simulink model "Model-Reglare"  (R2021b)
settings: Solver=ode45  StartTime=0.0  StopTime=1000  RelTol=1e-3  EnableMultiTasking=on
undefined symbols (not defined in the file): k, k1, k11, k12, k13, k2, k3, keta
libraries: slpidlib x8
(part 1 of 2)
settings Model: Creator=Nicoleta  LastModifiedBy=daria.chiriac
settings SolverCC: AlgebraicLoopSolver=TrustRegion
settings DataIOCC: LimitDataPoints=on  SaveFormat=Array  ReturnWorkspaceOutputs=off
settings OptimizationCC: LifeSpan=inf
settings DebuggingCC: SFUnexpectedBacktrackingDiag=warning  SFNoUnconditionalDefaultTransitionDiag=warning  SFExecutionAtInitializationDiag=none  SFMachineParentedDataDiag=warning  ArithmeticOperatorsInVariantConditions=warning
settings HardwareCC: ProdBitPerPointer=32  ProdBitPerSizeT=32  ProdBitPerPtrDiffT=32  ProdLargestAtomicFloat=None  ProdIntDivRoundTo=Undefined  ProdEndianess=Unspecified  ProdWordSize=32  ProdHWDeviceType=32-bit Generic
settings ModelReferenceCC: PropagateSignalLabelsOutOfModel=off
settings SFSimCC: SimUseLocalCustomCode=off  CustomCodeUndefinedFunction=UseInterfaceOnly
settings RTWCC: RTWUseLocalCustomCode=off
settings CodeAppCC: StateflowObjectComments=on
settings GRTTargetCC: TargetLangStandard=C89/C90 (ANSI)
settings ConfigComp: CovMetricSettings=dw  CovSaveCumulativeToWorkspaceVar=on  CovSaveSingleToWorkspaceVar=on  CovExternalEMLEnable=off

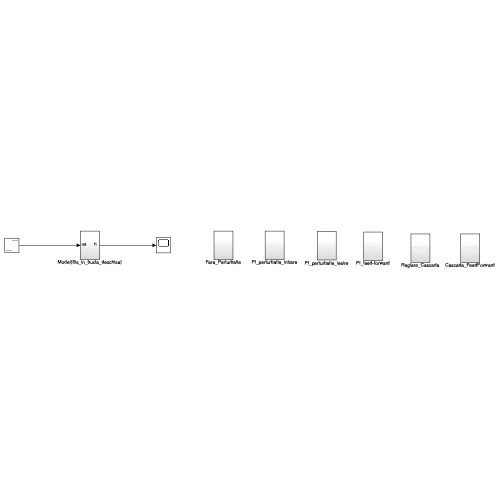
[thumbnail: Simulink's stored preview of the top-level diagram]
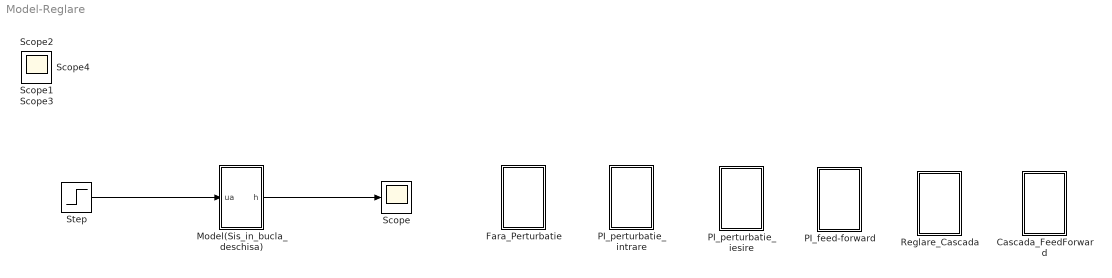
== system Model-Reglare ==
  Cascada_FeedForward : Subsystem
  Fara_Perturbatie : Subsystem
  Model(Sis_in_bucla_deschisa) : Subsystem
  PI_feed-forward : Subsystem
  PI_perturbatie_iesire : Subsystem
  PI_perturbatie_intrare : Subsystem
  Reglare_Cascada : Subsystem
  Scope{,1..4} (5 alike) : Scope
  Step : Step  After=5  SampleTime=0
  wires:
  Model(Sis_in_bucla_deschisa)/1("h ") -> Scope/1
  Step/1 -> Model(Sis_in_bucla_deschisa)/1("ua ")

== system Model-Reglare/Cascada_FeedForward ==
  Gain2 : Gain  Gain=1/3
  Gain3 : Gain  Gain=1/3
  PID Controller2 : slpidlib/PID Controller  Controller=PI  Form=Parallel  TimeDomain=Continuous-time  UseExternalTs=off  SampleTime=-1  IntegratorMethod=Forward Euler  FilterMethod=Forward Euler  ControllerParametersSource=internal  P=40  I=40/250  D=0  UseFilter=on  N=100  TunerSelectOption=Transfer Function Based (PID Tuner App)  InitialConditionSource=internal  InitialConditionForIntegrator=29.2  InitialConditionForFilter=0  DifferentiatorICPrevScaledInput=0  ExternalReset=none  TrackingMode=off  Kt=1  LimitOutput=off  SatLimitsSource=internal  UpperSaturationLimit=inf  LowerSaturationLimit=-inf  LinearizeAsGain=on  AntiWindupMode=none  Kb=1  POutMin=[]  POutMax=[]  IOutMin=[]  IOutMax=[]  DOutMin=[]  DOutMax=[]  NOutMin=[]  NOutMax=[]  SumOutMin=[]  SumOutMax=[]  SaturationOutMin=[]  SaturationOutMax=[]  PParamMin=[]  PParamMax=[]  IParamMin=[]  IParamMax=[]  DParamMin=[]  DParamMax=[]  NParamMin=[]  NParamMax=[]  KbParamMin=[]  KbParamMax=[]  KtParamMin=[]  KtParamMax=[]  KbOutMin=[]  KbOutMax=[]  KtOutMin=[]  KtOutMax=[]  IntegratorOutMin=[]  IntegratorOutMax=[]  FilterOutMin=[]  FilterOutMax=[]  SumI1OutMin=[]  SumI1OutMax=[]  SumI2OutMin=[]  SumI2OutMax=[]  SumI3OutMin=[]  SumI3OutMax=[]  SumI4OutMin=[]  SumI4OutMax=[]  SumDOutMin=[]  SumDOutMax=[]  DifferentiatorOutMin=[]  DifferentiatorOutMax=[]  FilterDiffOutCoefMin=[]  FilterDiffOutCoefMax=[]  ReciprocalOutMin=[]  ReciprocalOutMax=[]  SumDenOutMin=[]  SumDenOutMax=[]  SumNumOutMin=[]  SumNumOutMax=[]  DivideOutMin=[]  DivideOutMax=[]  UdiffTsProdOutMin=[]  UdiffTsProdOutMax=[]  NTsProdOutMin=[]  NTsProdOutMax=[]  UintegralTsProdOutMin=[]  UintegralTsProdOutMax=[]  UngainTsProdOutMin=[]  UngainTsProdOutMax=[]  FilterDenConstantOutDataTypeStr=Inherit: Inherit via back propagation  FilterDenConstantOutMin=[]  FilterDenConstantOutMax=[]  PCopyOutDataTypeStr=Inherit: Inherit via back propagation  PCopyOutMin=[]  PCopyOutMax=[]  NCopyOutDataTypeStr=Inherit: Inherit via back propagation  NCopyOutMin=[]  NCopyOutMax=[]  IntegratorContinuousStateAttributes=''  IntegratorStateMustResolveToSignalObject=off  IntegratorRTWStateStorageClass=Auto  FilterContinuousStateAttributes=''  FilterStateMustResolveToSignalObject=off  FilterRTWStateStorageClass=Auto  ParallelPVariant=InternalParameters  IdealPVariant=Disabled  IVariant=InternalParameters  DVariant=Disabled  IntegratorVariant=Continuous  SatVariant=Disabled  AWVariant=Passthrough  PCopyVariant=Disabled  TRVariant=Disabled  FdbkBlocksVariant=Forward  IdealPFdbkVariant=Disabled  SatFdbkVariant=Disabled  DerivativeFilterVariant=Disabled  NVariant=Disabled  NCopyVariant=Disabled_SignalSpec  FilterICVariant=Disabled  IntegratorICVariant=InternalICs  ExternalResetVariant=Disabled  TRSumVariant=Passthrough  SumFdbkVariant=Disabled  SumVariant=Sum_PI  TsampFilterVariant=InternalTs  TsampNgainVariant=Passthrough  TsampIntegralVariant=Passthrough  ExternalSaturationOutDataTypeStr=Inherit: Same as second input
  PID Controller3 : slpidlib/PID Controller  Controller=PI  Form=Parallel  TimeDomain=Continuous-time  UseExternalTs=off  SampleTime=-1  IntegratorMethod=Forward Euler  FilterMethod=Forward Euler  ControllerParametersSource=internal  P=0.07  I=1  D=0  UseFilter=on  N=100  TunerSelectOption=Transfer Function Based (PID Tuner App)  InitialConditionSource=internal  InitialConditionForIntegrator=5  InitialConditionForFilter=0  DifferentiatorICPrevScaledInput=0  ExternalReset=none  TrackingMode=off  Kt=1  LimitOutput=off  SatLimitsSource=internal  UpperSaturationLimit=inf  LowerSaturationLimit=-inf  LinearizeAsGain=on  AntiWindupMode=none  Kb=1  POutMin=[]  POutMax=[]  IOutMin=[]  IOutMax=[]  DOutMin=[]  DOutMax=[]  NOutMin=[]  NOutMax=[]  SumOutMin=[]  SumOutMax=[]  SaturationOutMin=[]  SaturationOutMax=[]  PParamMin=[]  PParamMax=[]  IParamMin=[]  IParamMax=[]  DParamMin=[]  DParamMax=[]  NParamMin=[]  NParamMax=[]  KbParamMin=[]  KbParamMax=[]  KtParamMin=[]  KtParamMax=[]  KbOutMin=[]  KbOutMax=[]  KtOutMin=[]  KtOutMax=[]  IntegratorOutMin=[]  IntegratorOutMax=[]  FilterOutMin=[]  FilterOutMax=[]  SumI1OutMin=[]  SumI1OutMax=[]  SumI2OutMin=[]  SumI2OutMax=[]  SumI3OutMin=[]  SumI3OutMax=[]  SumI4OutMin=[]  SumI4OutMax=[]  SumDOutMin=[]  SumDOutMax=[]  DifferentiatorOutMin=[]  DifferentiatorOutMax=[]  FilterDiffOutCoefMin=[]  FilterDiffOutCoefMax=[]  ReciprocalOutMin=[]  ReciprocalOutMax=[]  SumDenOutMin=[]  SumDenOutMax=[]  SumNumOutMin=[]  SumNumOutMax=[]  DivideOutMin=[]  DivideOutMax=[]  UdiffTsProdOutMin=[]  UdiffTsProdOutMax=[]  NTsProdOutMin=[]  NTsProdOutMax=[]  UintegralTsProdOutMin=[]  UintegralTsProdOutMax=[]  UngainTsProdOutMin=[]  UngainTsProdOutMax=[]  FilterDenConstantOutDataTypeStr=Inherit: Inherit via back propagation  FilterDenConstantOutMin=[]  FilterDenConstantOutMax=[]  PCopyOutDataTypeStr=Inherit: Inherit via back propagation  PCopyOutMin=[]  PCopyOutMax=[]  NCopyOutDataTypeStr=Inherit: Inherit via back propagation  NCopyOutMin=[]  NCopyOutMax=[]  IntegratorContinuousStateAttributes=''  IntegratorStateMustResolveToSignalObject=off  IntegratorRTWStateStorageClass=Auto  FilterContinuousStateAttributes=''  FilterStateMustResolveToSignalObject=off  FilterRTWStateStorageClass=Auto  ParallelPVariant=InternalParameters  IdealPVariant=Disabled  IVariant=InternalParameters  DVariant=Disabled  IntegratorVariant=Continuous  SatVariant=Disabled  AWVariant=Passthrough  PCopyVariant=Disabled  TRVariant=Disabled  FdbkBlocksVariant=Forward  IdealPFdbkVariant=Disabled  SatFdbkVariant=Disabled  DerivativeFilterVariant=Disabled  NVariant=Disabled  NCopyVariant=Disabled_SignalSpec  FilterICVariant=Disabled  IntegratorICVariant=InternalICs  ExternalResetVariant=Disabled  TRSumVariant=Passthrough  SumFdbkVariant=Disabled  SumVariant=Sum_PI  TsampFilterVariant=InternalTs  TsampNgainVariant=Passthrough  TsampIntegralVariant=Passthrough  ExternalSaturationOutDataTypeStr=Inherit: Same as second input
  Scope5 : Scope
  Scope6 : Scope
  Sum2 : Sum  Inputs=|+-
  Sum3 : Sum  Inputs=++-
  h*1 : Step  Before=10.5  After=13  SampleTime=0
  modelproiect 1 : Subsystem
  wires:
  modelproiect 1/3(q1) -> Sum3/3
  Gain3/1 -> Sum2/2
  PID Controller3/1 -> modelproiect 1/1("ua ")
  h*1/1 -> Gain2/1
  Gain2/1 -> Sum2/1
  PID Controller2/1 -> Sum3/2
  modelproiect 1/2(Perturbatie) -> Sum3/1, Scope6/1
  Sum3/1 -> PID Controller3/1
  Sum2/1 -> PID Controller2/1
  modelproiect 1/1("h ") -> Gain3/1, Scope5/1

== system Model-Reglare/Fara_Perturbatie ==
  Gain : Gain  Gain=1/3
  Gain1 : Gain  Gain=1/3
  PID Controller1 : slpidlib/PID Controller  Controller=PI  Form=Parallel  TimeDomain=Continuous-time  UseExternalTs=off  SampleTime=-1  IntegratorMethod=Forward Euler  FilterMethod=Forward Euler  ControllerParametersSource=internal  P=2.395  I=2.395/160  D=0  UseFilter=on  N=100  TunerSelectOption=Transfer Function Based (PID Tuner App)  InitialConditionSource=internal  InitialConditionForIntegrator=5  InitialConditionForFilter=0  DifferentiatorICPrevScaledInput=0  ExternalReset=none  TrackingMode=off  Kt=1  LimitOutput=off  SatLimitsSource=internal  UpperSaturationLimit=inf  LowerSaturationLimit=-inf  LinearizeAsGain=on  AntiWindupMode=none  Kb=1  POutMin=[]  POutMax=[]  IOutMin=[]  IOutMax=[]  DOutMin=[]  DOutMax=[]  NOutMin=[]  NOutMax=[]  SumOutMin=[]  SumOutMax=[]  SaturationOutMin=[]  SaturationOutMax=[]  PParamMin=[]  PParamMax=[]  IParamMin=[]  IParamMax=[]  DParamMin=[]  DParamMax=[]  NParamMin=[]  NParamMax=[]  KbParamMin=[]  KbParamMax=[]  KtParamMin=[]  KtParamMax=[]  KbOutMin=[]  KbOutMax=[]  KtOutMin=[]  KtOutMax=[]  IntegratorOutMin=[]  IntegratorOutMax=[]  FilterOutMin=[]  FilterOutMax=[]  SumI1OutMin=[]  SumI1OutMax=[]  SumI2OutMin=[]  SumI2OutMax=[]  SumI3OutMin=[]  SumI3OutMax=[]  SumI4OutMin=[]  SumI4OutMax=[]  SumDOutMin=[]  SumDOutMax=[]  DifferentiatorOutMin=[]  DifferentiatorOutMax=[]  FilterDiffOutCoefMin=[]  FilterDiffOutCoefMax=[]  ReciprocalOutMin=[]  ReciprocalOutMax=[]  SumDenOutMin=[]  SumDenOutMax=[]  SumNumOutMin=[]  SumNumOutMax=[]  DivideOutMin=[]  DivideOutMax=[]  UdiffTsProdOutMin=[]  UdiffTsProdOutMax=[]  NTsProdOutMin=[]  NTsProdOutMax=[]  UintegralTsProdOutMin=[]  UintegralTsProdOutMax=[]  UngainTsProdOutMin=[]  UngainTsProdOutMax=[]  FilterDenConstantOutDataTypeStr=Inherit: Inherit via back propagation  FilterDenConstantOutMin=[]  FilterDenConstantOutMax=[]  PCopyOutDataTypeStr=Inherit: Inherit via back propagation  PCopyOutMin=[]  PCopyOutMax=[]  NCopyOutDataTypeStr=Inherit: Inherit via back propagation  NCopyOutMin=[]  NCopyOutMax=[]  IntegratorContinuousStateAttributes=''  IntegratorStateMustResolveToSignalObject=off  IntegratorRTWStateStorageClass=Auto  FilterContinuousStateAttributes=''  FilterStateMustResolveToSignalObject=off  FilterRTWStateStorageClass=Auto  ParallelPVariant=InternalParameters  IdealPVariant=Disabled  IVariant=InternalParameters  DVariant=Disabled  IntegratorVariant=Continuous  SatVariant=Disabled  AWVariant=Passthrough  PCopyVariant=Disabled  TRVariant=Disabled  FdbkBlocksVariant=Forward  IdealPFdbkVariant=Disabled  SatFdbkVariant=Disabled  DerivativeFilterVariant=Disabled  NVariant=Disabled  NCopyVariant=Disabled_SignalSpec  FilterICVariant=Disabled  IntegratorICVariant=InternalICs  ExternalResetVariant=Disabled  TRSumVariant=Passthrough  SumFdbkVariant=Disabled  SumVariant=Sum_PI  TsampFilterVariant=InternalTs  TsampNgainVariant=Passthrough  TsampIntegralVariant=Passthrough  ExternalSaturationOutDataTypeStr=Inherit: Same as second input
  Sistem in bucla deschisa 1 : Subsystem
  Sum : Sum  Inputs=|+-
  "comanda " : Scope
  "h " : Scope
  h* : Step  Before=10.5  After=13  SampleTime=0
  wires:
  Gain/1 -> Sum/2
  Sum/1 -> PID Controller1/1
  Gain1/1 -> Sum/1
  h*/1 -> Gain1/1
  Sistem in bucla deschisa 1/1("h ") -> Gain/1, "h "/1
  PID Controller1/1 -> Sistem in bucla deschisa 1/1("ua "), "comanda "/1

== system Model-Reglare/Model(Sis_in_bucla_deschisa) ==
  "ua " : Inport
  "Amplificator " : Subsystem
  "Filtru " : Subsystem
  Motor : Subsystem
  "Randament " : Subsystem
  "Rezervor " : Subsystem
  Scope : Scope
  Scope1 : Scope
  "curent " : Subsystem
  "pompa " : Subsystem
  "h " : Outport  VectorParamsAs1DForOutWhenUnconnected=off
  wires:
  "Filtru "/1(q_f) -> Scope1/1, "Randament "/1(q), "curent "/1(q), "Rezervor "/1("qi ")
  Motor/1(kn) -> "pompa "/1(kn)
  "Rezervor "/1(h) -> Scope/1, "curent "/3("h "), "pompa "/2("h "), "h "/1
  "Randament "/1("eta ") -> "curent "/2(eta)
  "pompa "/1("q ") -> "Filtru "/1("qi ")
  "Amplificator "/1("um ") -> Motor/1("um "), "Randament "/2("um "), "curent "/4(um)
  "curent "/1("im ") -> Motor/2("im ")
  "ua "/1 -> "Amplificator "/1("ua ")

== system Model-Reglare/PI_feed-forward ==
  Gain : Gain  Gain=1/3
  Gain1 : Gain  Gain=1/3
  Gain2 : Gain  Gain=0.1
  Model(Sis_in_bucla_deschisa) : Subsystem
  PID Controller : slpidlib/PID Controller  Controller=PI  Form=Parallel  TimeDomain=Continuous-time  UseExternalTs=off  SampleTime=-1  IntegratorMethod=Forward Euler  FilterMethod=Forward Euler  ControllerParametersSource=internal  P=2.395  I=2.395/160  D=0  UseFilter=on  N=100  TunerSelectOption=Transfer Function Based (PID Tuner App)  InitialConditionSource=internal  InitialConditionForIntegrator=5  InitialConditionForFilter=0  DifferentiatorICPrevScaledInput=0  ExternalReset=none  TrackingMode=off  Kt=1  LimitOutput=off  SatLimitsSource=internal  UpperSaturationLimit=inf  LowerSaturationLimit=-inf  LinearizeAsGain=on  AntiWindupMode=none  Kb=1  POutMin=[]  POutMax=[]  IOutMin=[]  IOutMax=[]  DOutMin=[]  DOutMax=[]  NOutMin=[]  NOutMax=[]  SumOutMin=[]  SumOutMax=[]  SaturationOutMin=[]  SaturationOutMax=[]  PParamMin=[]  PParamMax=[]  IParamMin=[]  IParamMax=[]  DParamMin=[]  DParamMax=[]  NParamMin=[]  NParamMax=[]  KbParamMin=[]  KbParamMax=[]  KtParamMin=[]  KtParamMax=[]  KbOutMin=[]  KbOutMax=[]  KtOutMin=[]  KtOutMax=[]  IntegratorOutMin=[]  IntegratorOutMax=[]  FilterOutMin=[]  FilterOutMax=[]  SumI1OutMin=[]  SumI1OutMax=[]  SumI2OutMin=[]  SumI2OutMax=[]  SumI3OutMin=[]  SumI3OutMax=[]  SumI4OutMin=[]  SumI4OutMax=[]  SumDOutMin=[]  SumDOutMax=[]  DifferentiatorOutMin=[]  DifferentiatorOutMax=[]  FilterDiffOutCoefMin=[]  FilterDiffOutCoefMax=[]  ReciprocalOutMin=[]  ReciprocalOutMax=[]  SumDenOutMin=[]  SumDenOutMax=[]  SumNumOutMin=[]  SumNumOutMax=[]  DivideOutMin=[]  DivideOutMax=[]  UdiffTsProdOutMin=[]  UdiffTsProdOutMax=[]  NTsProdOutMin=[]  NTsProdOutMax=[]  UintegralTsProdOutMin=[]  UintegralTsProdOutMax=[]  UngainTsProdOutMin=[]  UngainTsProdOutMax=[]  FilterDenConstantOutDataTypeStr=Inherit: Inherit via back propagation  FilterDenConstantOutMin=[]  FilterDenConstantOutMax=[]  PCopyOutDataTypeStr=Inherit: Inherit via back propagation  PCopyOutMin=[]  PCopyOutMax=[]  NCopyOutDataTypeStr=Inherit: Inherit via back propagation  NCopyOutMin=[]  NCopyOutMax=[]  IntegratorContinuousStateAttributes=''  IntegratorStateMustResolveToSignalObject=off  IntegratorRTWStateStorageClass=Auto  FilterContinuousStateAttributes=''  FilterStateMustResolveToSignalObject=off  FilterRTWStateStorageClass=Auto  ParallelPVariant=InternalParameters  IdealPVariant=Disabled  IVariant=InternalParameters  DVariant=Disabled  IntegratorVariant=Continuous  SatVariant=Disabled  AWVariant=Passthrough  PCopyVariant=Disabled  TRVariant=Disabled  FdbkBlocksVariant=Forward  IdealPFdbkVariant=Disabled  SatFdbkVariant=Disabled  DerivativeFilterVariant=Disabled  NVariant=Disabled  NCopyVariant=Disabled_SignalSpec  FilterICVariant=Disabled  IntegratorICVariant=InternalICs  ExternalResetVariant=Disabled  TRSumVariant=Passthrough  SumFdbkVariant=Disabled  SumVariant=Sum_PI  TsampFilterVariant=InternalTs  TsampNgainVariant=Passthrough  TsampIntegralVariant=Passthrough  ExternalSaturationOutDataTypeStr=Inherit: Same as second input
  Sum : Sum  Inputs=|+-
  Sum1 : Sum  Inputs=|++
  "comanda " : Scope
  "h " : Scope
  h* : Step  Before=10.5  After=13  SampleTime=0
  wires:
  Gain2/1 -> Sum1/2
  Sum/1 -> PID Controller/1
  Gain1/1 -> Sum/1
  h*/1 -> Gain1/1
  PID Controller/1 -> Sum1/1
  Model(Sis_in_bucla_deschisa)/2("Perturbatie ") -> Gain2/1
  Model(Sis_in_bucla_deschisa)/1("h ") -> Gain/1, "h "/1
  Gain/1 -> Sum/2
  Sum1/1 -> "comanda "/1, Model(Sis_in_bucla_deschisa)/1("ua ")

== system Model-Reglare/PI_perturbatie_iesire ==
  Gain : Gain  Gain=1/3
  Gain1 : Gain  Gain=1/3
  "Model_Modificat " : Subsystem
  PID Controller : slpidlib/PID Controller  Controller=PI  Form=Parallel  TimeDomain=Continuous-time  UseExternalTs=off  SampleTime=-1  IntegratorMethod=Forward Euler  FilterMethod=Forward Euler  ControllerParametersSource=internal  P=2.395  I=2.395/160  D=0  UseFilter=on  N=100  TunerSelectOption=Transfer Function Based (PID Tuner App)  InitialConditionSource=internal  InitialConditionForIntegrator=5  InitialConditionForFilter=0  DifferentiatorICPrevScaledInput=0  ExternalReset=none  TrackingMode=off  Kt=1  LimitOutput=off  SatLimitsSource=internal  UpperSaturationLimit=inf  LowerSaturationLimit=-inf  LinearizeAsGain=on  AntiWindupMode=none  Kb=1  POutMin=[]  POutMax=[]  IOutMin=[]  IOutMax=[]  DOutMin=[]  DOutMax=[]  NOutMin=[]  NOutMax=[]  SumOutMin=[]  SumOutMax=[]  SaturationOutMin=[]  SaturationOutMax=[]  PParamMin=[]  PParamMax=[]  IParamMin=[]  IParamMax=[]  DParamMin=[]  DParamMax=[]  NParamMin=[]  NParamMax=[]  KbParamMin=[]  KbParamMax=[]  KtParamMin=[]  KtParamMax=[]  KbOutMin=[]  KbOutMax=[]  KtOutMin=[]  KtOutMax=[]  IntegratorOutMin=[]  IntegratorOutMax=[]  FilterOutMin=[]  FilterOutMax=[]  SumI1OutMin=[]  SumI1OutMax=[]  SumI2OutMin=[]  SumI2OutMax=[]  SumI3OutMin=[]  SumI3OutMax=[]  SumI4OutMin=[]  SumI4OutMax=[]  SumDOutMin=[]  SumDOutMax=[]  DifferentiatorOutMin=[]  DifferentiatorOutMax=[]  FilterDiffOutCoefMin=[]  FilterDiffOutCoefMax=[]  ReciprocalOutMin=[]  ReciprocalOutMax=[]  SumDenOutMin=[]  SumDenOutMax=[]  SumNumOutMin=[]  SumNumOutMax=[]  DivideOutMin=[]  DivideOutMax=[]  UdiffTsProdOutMin=[]  UdiffTsProdOutMax=[]  NTsProdOutMin=[]  NTsProdOutMax=[]  UintegralTsProdOutMin=[]  UintegralTsProdOutMax=[]  UngainTsProdOutMin=[]  UngainTsProdOutMax=[]  FilterDenConstantOutDataTypeStr=Inherit: Inherit via back propagation  FilterDenConstantOutMin=[]  FilterDenConstantOutMax=[]  PCopyOutDataTypeStr=Inherit: Inherit via back propagation  PCopyOutMin=[]  PCopyOutMax=[]  NCopyOutDataTypeStr=Inherit: Inherit via back propagation  NCopyOutMin=[]  NCopyOutMax=[]  IntegratorContinuousStateAttributes=''  IntegratorStateMustResolveToSignalObject=off  IntegratorRTWStateStorageClass=Auto  FilterContinuousStateAttributes=''  FilterStateMustResolveToSignalObject=off  FilterRTWStateStorageClass=Auto  ParallelPVariant=InternalParameters  IdealPVariant=Disabled  IVariant=InternalParameters  DVariant=Disabled  IntegratorVariant=Continuous  SatVariant=Disabled  AWVariant=Passthrough  PCopyVariant=Disabled  TRVariant=Disabled  FdbkBlocksVariant=Forward  IdealPFdbkVariant=Disabled  SatFdbkVariant=Disabled  DerivativeFilterVariant=Disabled  NVariant=Disabled  NCopyVariant=Disabled_SignalSpec  FilterICVariant=Disabled  IntegratorICVariant=InternalICs  ExternalResetVariant=Disabled  TRSumVariant=Passthrough  SumFdbkVariant=Disabled  SumVariant=Sum_PI  TsampFilterVariant=InternalTs  TsampNgainVariant=Passthrough  TsampIntegralVariant=Passthrough  ExternalSaturationOutDataTypeStr=Inherit: Same as second input
  Sum : Sum  Inputs=|+-
  "comanda " : Scope
  "h " : Scope
  h* : Step  Before=10.5  After=13  SampleTime=0
  wires:
  Sum/1 -> PID Controller/1
  h*/1 -> Gain1/1
  "Model_Modificat "/1("h ") -> Gain/1, "h "/1
  PID Controller/1 -> "comanda "/1, "Model_Modificat "/1("ua ")
  Gain/1 -> Sum/2
  Gain1/1 -> Sum/1

== system Model-Reglare/PI_perturbatie_intrare ==
  Gain : Gain  Gain=1/3
  Gain1 : Gain  Gain=1/3
  "Model_cu_perturbatie " : Subsystem
  PID Controller : slpidlib/PID Controller  Controller=PI  Form=Parallel  TimeDomain=Continuous-time  UseExternalTs=off  SampleTime=-1  IntegratorMethod=Forward Euler  FilterMethod=Forward Euler  ControllerParametersSource=internal  P=2.395  I=2.395/160  D=0  UseFilter=on  N=100  TunerSelectOption=Transfer Function Based (PID Tuner App)  InitialConditionSource=internal  InitialConditionForIntegrator=5  InitialConditionForFilter=0  DifferentiatorICPrevScaledInput=0  ExternalReset=none  TrackingMode=off  Kt=1  LimitOutput=off  SatLimitsSource=internal  UpperSaturationLimit=inf  LowerSaturationLimit=-inf  LinearizeAsGain=on  AntiWindupMode=none  Kb=1  POutMin=[]  POutMax=[]  IOutMin=[]  IOutMax=[]  DOutMin=[]  DOutMax=[]  NOutMin=[]  NOutMax=[]  SumOutMin=[]  SumOutMax=[]  SaturationOutMin=[]  SaturationOutMax=[]  PParamMin=[]  PParamMax=[]  IParamMin=[]  IParamMax=[]  DParamMin=[]  DParamMax=[]  NParamMin=[]  NParamMax=[]  KbParamMin=[]  KbParamMax=[]  KtParamMin=[]  KtParamMax=[]  KbOutMin=[]  KbOutMax=[]  KtOutMin=[]  KtOutMax=[]  IntegratorOutMin=[]  IntegratorOutMax=[]  FilterOutMin=[]  FilterOutMax=[]  SumI1OutMin=[]  SumI1OutMax=[]  SumI2OutMin=[]  SumI2OutMax=[]  SumI3OutMin=[]  SumI3OutMax=[]  SumI4OutMin=[]  SumI4OutMax=[]  SumDOutMin=[]  SumDOutMax=[]  DifferentiatorOutMin=[]  DifferentiatorOutMax=[]  FilterDiffOutCoefMin=[]  FilterDiffOutCoefMax=[]  ReciprocalOutMin=[]  ReciprocalOutMax=[]  SumDenOutMin=[]  SumDenOutMax=[]  SumNumOutMin=[]  SumNumOutMax=[]  DivideOutMin=[]  DivideOutMax=[]  UdiffTsProdOutMin=[]  UdiffTsProdOutMax=[]  NTsProdOutMin=[]  NTsProdOutMax=[]  UintegralTsProdOutMin=[]  UintegralTsProdOutMax=[]  UngainTsProdOutMin=[]  UngainTsProdOutMax=[]  FilterDenConstantOutDataTypeStr=Inherit: Inherit via back propagation  FilterDenConstantOutMin=[]  FilterDenConstantOutMax=[]  PCopyOutDataTypeStr=Inherit: Inherit via back propagation  PCopyOutMin=[]  PCopyOutMax=[]  NCopyOutDataTypeStr=Inherit: Inherit via back propagation  NCopyOutMin=[]  NCopyOutMax=[]  IntegratorContinuousStateAttributes=''  IntegratorStateMustResolveToSignalObject=off  IntegratorRTWStateStorageClass=Auto  FilterContinuousStateAttributes=''  FilterStateMustResolveToSignalObject=off  FilterRTWStateStorageClass=Auto  ParallelPVariant=InternalParameters  IdealPVariant=Disabled  IVariant=InternalParameters  DVariant=Disabled  IntegratorVariant=Continuous  SatVariant=Disabled  AWVariant=Passthrough  PCopyVariant=Disabled  TRVariant=Disabled  FdbkBlocksVariant=Forward  IdealPFdbkVariant=Disabled  SatFdbkVariant=Disabled  DerivativeFilterVariant=Disabled  NVariant=Disabled  NCopyVariant=Disabled_SignalSpec  FilterICVariant=Disabled  IntegratorICVariant=InternalICs  ExternalResetVariant=Disabled  TRSumVariant=Passthrough  SumFdbkVariant=Disabled  SumVariant=Sum_PI  TsampFilterVariant=InternalTs  TsampNgainVariant=Passthrough  TsampIntegralVariant=Passthrough  ExternalSaturationOutDataTypeStr=Inherit: Same as second input
  Sum : Sum  Inputs=|+-
  "comanda " : Scope
  "h " : Scope
  h* : Step  Before=10.5  After=13  SampleTime=0
  wires:
  "Model_cu_perturbatie "/1("h ") -> Gain/1, "h "/1
  Gain1/1 -> Sum/1
  Sum/1 -> PID Controller/1
  Gain/1 -> Sum/2
  PID Controller/1 -> "Model_cu_perturbatie "/1("ua "), "comanda "/1
  h*/1 -> Gain1/1

== system Model-Reglare/Reglare_Cascada ==
  Gain2 : Gain  Gain=1/3
  Gain3 : Gain  Gain=1/3
  PID Controller2 : slpidlib/PID Controller  Controller=PI  Form=Parallel  TimeDomain=Continuous-time  UseExternalTs=off  SampleTime=-1  IntegratorMethod=Forward Euler  FilterMethod=Forward Euler  ControllerParametersSource=internal  P=40  I=40/250  D=0  UseFilter=on  N=100  TunerSelectOption=Transfer Function Based (PID Tuner App)  InitialConditionSource=internal  InitialConditionForIntegrator=29.2  InitialConditionForFilter=0  DifferentiatorICPrevScaledInput=0  ExternalReset=none  TrackingMode=off  Kt=1  LimitOutput=off  SatLimitsSource=internal  UpperSaturationLimit=inf  LowerSaturationLimit=-inf  LinearizeAsGain=on  AntiWindupMode=none  Kb=1  POutMin=[]  POutMax=[]  IOutMin=[]  IOutMax=[]  DOutMin=[]  DOutMax=[]  NOutMin=[]  NOutMax=[]  SumOutMin=[]  SumOutMax=[]  SaturationOutMin=[]  SaturationOutMax=[]  PParamMin=[]  PParamMax=[]  IParamMin=[]  IParamMax=[]  DParamMin=[]  DParamMax=[]  NParamMin=[]  NParamMax=[]  KbParamMin=[]  KbParamMax=[]  KtParamMin=[]  KtParamMax=[]  KbOutMin=[]  KbOutMax=[]  KtOutMin=[]  KtOutMax=[]  IntegratorOutMin=[]  IntegratorOutMax=[]  FilterOutMin=[]  FilterOutMax=[]  SumI1OutMin=[]  SumI1OutMax=[]  SumI2OutMin=[]  SumI2OutMax=[]  SumI3OutMin=[]  SumI3OutMax=[]  SumI4OutMin=[]  SumI4OutMax=[]  SumDOutMin=[]  SumDOutMax=[]  DifferentiatorOutMin=[]  DifferentiatorOutMax=[]  FilterDiffOutCoefMin=[]  FilterDiffOutCoefMax=[]  ReciprocalOutMin=[]  ReciprocalOutMax=[]  SumDenOutMin=[]  SumDenOutMax=[]  SumNumOutMin=[]  SumNumOutMax=[]  DivideOutMin=[]  DivideOutMax=[]  UdiffTsProdOutMin=[]  UdiffTsProdOutMax=[]  NTsProdOutMin=[]  NTsProdOutMax=[]  UintegralTsProdOutMin=[]  UintegralTsProdOutMax=[]  UngainTsProdOutMin=[]  UngainTsProdOutMax=[]  FilterDenConstantOutDataTypeStr=Inherit: Inherit via back propagation  FilterDenConstantOutMin=[]  FilterDenConstantOutMax=[]  PCopyOutDataTypeStr=Inherit: Inherit via back propagation  PCopyOutMin=[]  PCopyOutMax=[]  NCopyOutDataTypeStr=Inherit: Inherit via back propagation  NCopyOutMin=[]  NCopyOutMax=[]  IntegratorContinuousStateAttributes=''  IntegratorStateMustResolveToSignalObject=off  IntegratorRTWStateStorageClass=Auto  FilterContinuousStateAttributes=''  FilterStateMustResolveToSignalObject=off  FilterRTWStateStorageClass=Auto  ParallelPVariant=InternalParameters  IdealPVariant=Disabled  IVariant=InternalParameters  DVariant=Disabled  IntegratorVariant=Continuous  SatVariant=Disabled  AWVariant=Passthrough  PCopyVariant=Disabled  TRVariant=Disabled  FdbkBlocksVariant=Forward  IdealPFdbkVariant=Disabled  SatFdbkVariant=Disabled  DerivativeFilterVariant=Disabled  NVariant=Disabled  NCopyVariant=Disabled_SignalSpec  FilterICVariant=Disabled  IntegratorICVariant=InternalICs  ExternalResetVariant=Disabled  TRSumVariant=Passthrough  SumFdbkVariant=Disabled  SumVariant=Sum_PI  TsampFilterVariant=InternalTs  TsampNgainVariant=Passthrough  TsampIntegralVariant=Passthrough  ExternalSaturationOutDataTypeStr=Inherit: Same as second input
  PID Controller3 : slpidlib/PID Controller  Controller=PI  Form=Parallel  TimeDomain=Continuous-time  UseExternalTs=off  SampleTime=-1  IntegratorMethod=Forward Euler  FilterMethod=Forward Euler  ControllerParametersSource=internal  P=0.07  I=1  D=0  UseFilter=on  N=100  TunerSelectOption=Transfer Function Based (PID Tuner App)  InitialConditionSource=internal  InitialConditionForIntegrator=5  InitialConditionForFilter=0  DifferentiatorICPrevScaledInput=0  ExternalReset=none  TrackingMode=off  Kt=1  LimitOutput=off  SatLimitsSource=internal  UpperSaturationLimit=inf  LowerSaturationLimit=-inf  LinearizeAsGain=on  AntiWindupMode=none  Kb=1  POutMin=[]  POutMax=[]  IOutMin=[]  IOutMax=[]  DOutMin=[]  DOutMax=[]  NOutMin=[]  NOutMax=[]  SumOutMin=[]  SumOutMax=[]  SaturationOutMin=[]  SaturationOutMax=[]  PParamMin=[]  PParamMax=[]  IParamMin=[]  IParamMax=[]  DParamMin=[]  DParamMax=[]  NParamMin=[]  NParamMax=[]  KbParamMin=[]  KbParamMax=[]  KtParamMin=[]  KtParamMax=[]  KbOutMin=[]  KbOutMax=[]  KtOutMin=[]  KtOutMax=[]  IntegratorOutMin=[]  IntegratorOutMax=[]  FilterOutMin=[]  FilterOutMax=[]  SumI1OutMin=[]  SumI1OutMax=[]  SumI2OutMin=[]  SumI2OutMax=[]  SumI3OutMin=[]  SumI3OutMax=[]  SumI4OutMin=[]  SumI4OutMax=[]  SumDOutMin=[]  SumDOutMax=[]  DifferentiatorOutMin=[]  DifferentiatorOutMax=[]  FilterDiffOutCoefMin=[]  FilterDiffOutCoefMax=[]  ReciprocalOutMin=[]  ReciprocalOutMax=[]  SumDenOutMin=[]  SumDenOutMax=[]  SumNumOutMin=[]  SumNumOutMax=[]  DivideOutMin=[]  DivideOutMax=[]  UdiffTsProdOutMin=[]  UdiffTsProdOutMax=[]  NTsProdOutMin=[]  NTsProdOutMax=[]  UintegralTsProdOutMin=[]  UintegralTsProdOutMax=[]  UngainTsProdOutMin=[]  UngainTsProdOutMax=[]  FilterDenConstantOutDataTypeStr=Inherit: Inherit via back propagation  FilterDenConstantOutMin=[]  FilterDenConstantOutMax=[]  PCopyOutDataTypeStr=Inherit: Inherit via back propagation  PCopyOutMin=[]  PCopyOutMax=[]  NCopyOutDataTypeStr=Inherit: Inherit via back propagation  NCopyOutMin=[]  NCopyOutMax=[]  IntegratorContinuousStateAttributes=''  IntegratorStateMustResolveToSignalObject=off  IntegratorRTWStateStorageClass=Auto  FilterContinuousStateAttributes=''  FilterStateMustResolveToSignalObject=off  FilterRTWStateStorageClass=Auto  ParallelPVariant=InternalParameters  IdealPVariant=Disabled  IVariant=InternalParameters  DVariant=Disabled  IntegratorVariant=Continuous  SatVariant=Disabled  AWVariant=Passthrough  PCopyVariant=Disabled  TRVariant=Disabled  FdbkBlocksVariant=Forward  IdealPFdbkVariant=Disabled  SatFdbkVariant=Disabled  DerivativeFilterVariant=Disabled  NVariant=Disabled  NCopyVariant=Disabled_SignalSpec  FilterICVariant=Disabled  IntegratorICVariant=InternalICs  ExternalResetVariant=Disabled  TRSumVariant=Passthrough  SumFdbkVariant=Disabled  SumVariant=Sum_PI  TsampFilterVariant=InternalTs  TsampNgainVariant=Passthrough  TsampIntegralVariant=Passthrough  ExternalSaturationOutDataTypeStr=Inherit: Same as second input
  Scope5 : Scope
  Scope6 : Scope
  Sum2 : Sum  Inputs=|+-
  Sum3 : Sum  Inputs=|+-
  h*1 : Step  Before=10.5  After=13  SampleTime=0
  "modelproiect " : Subsystem
  wires:
  h*1/1 -> Gain2/1
  "modelproiect "/2(Perturbatie) -> Scope6/1
  Gain2/1 -> Sum2/1
  PID Controller3/1 -> "modelproiect "/1("ua ")
  Gain3/1 -> Sum2/2
  Sum2/1 -> PID Controller2/1
  Sum3/1 -> PID Controller3/1
  "modelproiect "/1("h ") -> Gain3/1, Scope5/1
  PID Controller2/1 -> Sum3/1
  "modelproiect "/3(q1) -> Sum3/2

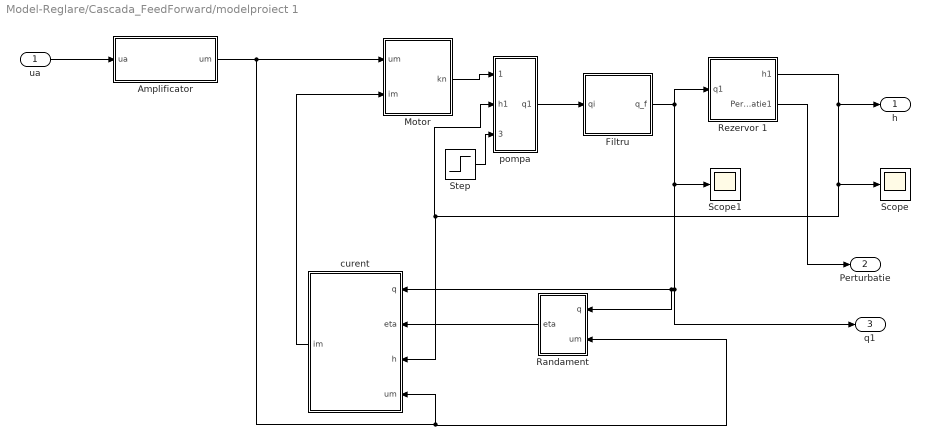
== system Model-Reglare/Cascada_FeedForward/modelproiect 1 ==
  "ua " : Inport
  "Amplificator " : Subsystem
  "Filtru " : Subsystem
  Motor : Subsystem
  "Randament " : Subsystem
  Rezervor 1 : Subsystem
  Scope : Scope
  Scope1 : Scope
  Step : Step  Time=300  After=k  SampleTime=0
  "curent " : Subsystem
  "pompa " : Subsystem
  "h " : Outport  VectorParamsAs1DForOutWhenUnconnected=off
  Perturbatie : Outport  Port=2  VectorParamsAs1DForOutWhenUnconnected=off
  q1 : Outport  Port=3  VectorParamsAs1DForOutWhenUnconnected=off
  wires:
  "Amplificator "/1("um ") -> Motor/1("um "), "Randament "/2("um "), "curent "/4(um)
  "curent "/1("im ") -> Motor/2("im ")
  Step/1 -> "pompa "/3(perturbatie k)
  Rezervor 1/1(h1) -> Scope/1, "pompa "/2(h1), "curent "/3("h "), "h "/1
  "pompa "/1(q1) -> "Filtru "/1("qi ")
  "Randament "/1("eta ") -> "curent "/2(eta)
  Motor/1(kn) -> "pompa "/1(kn1)
  "Filtru "/1(q_f) -> Rezervor 1/1(q1), Scope1/1, q1/1, "Randament "/1(q), "curent "/1(q)
  "ua "/1 -> "Amplificator "/1("ua ")
  Rezervor 1/2(Perturbatie1) -> Perturbatie/1

== system Model-Reglare/Fara_Perturbatie/Sistem in bucla deschisa 1 ==
  "ua " : Inport
  "Amplificator " : Subsystem
  "Filtru " : Subsystem
  Motor : Subsystem
  "Randament " : Subsystem
  "Rezervor " : Subsystem
  Scope : Scope
  Scope1 : Scope
  "curent " : Subsystem
  "pompa " : Subsystem
  "h " : Outport  VectorParamsAs1DForOutWhenUnconnected=off
  wires:
  "Filtru "/1(q_f) -> Scope1/1, "Randament "/1(q), "curent "/1(q), "Rezervor "/1("qi ")
  Motor/1(kn) -> "pompa "/1(kn)
  "Rezervor "/1(h) -> Scope/1, "curent "/3("h "), "pompa "/2("h "), "h "/1
  "Randament "/1("eta ") -> "curent "/2(eta)
  "pompa "/1("q ") -> "Filtru "/1("qi ")
  "Amplificator "/1("um ") -> Motor/1("um "), "Randament "/2("um "), "curent "/4(um)
  "curent "/1("im ") -> Motor/2("im ")
  "ua "/1 -> "Amplificator "/1("ua ")

== system Model-Reglare/Model(Sis_in_bucla_deschisa)/Amplificator  ==
  "ua " : Inport
  Constant : Constant  Value=8.1
  Gain : Gain  Gain=2.2
  Gain1 : Gain  Gain=2.2
  Gain2 : Gain  Gain=5
  Saturation : Saturate  UpperLimit=22  LowerLimit=0
  Sum : Sum  Inputs=|+-
  Sum1 : Sum  Inputs=|++
  Switch : Switch  Criteria=u2 > Threshold  Threshold=8.1
  "um " : Outport  VectorParamsAs1DForOutWhenUnconnected=off
  wires:
  Saturation/1 -> "um "/1
  Switch/1 -> Saturation/1
  Constant/1 -> Sum/2
  Sum/1 -> Gain2/1
  Sum1/1 -> Switch/1
  Gain1/1 -> Sum1/1
  Gain/1 -> Switch/3
  "ua "/1 -> Switch/2, Gain/1, Sum/1, Gain1/1
  Gain2/1 -> Sum1/2

== system Model-Reglare/Model(Sis_in_bucla_deschisa)/Filtru  ==
  "qi " : Inport
  Integrator : Integrator
  Sum : Sum  Inputs=|+-
  q_f : Outport  VectorParamsAs1DForOutWhenUnconnected=off
  wires:
  "qi "/1 -> Sum/1
  Sum/1 -> Integrator/1
  Integrator/1 -> Sum/2, q_f/1

== system Model-Reglare/Model(Sis_in_bucla_deschisa)/Motor ==
  "um " : Inport
  "im " : Inport  Port=2
  Add : Sum  Inputs=+-
  Rm : Gain  Gain=3
  kn : Outport  VectorParamsAs1DForOutWhenUnconnected=off
  wires:
  "um "/1 -> Add/1
  "im "/1 -> Rm/1
  Add/1 -> kn/1
  Rm/1 -> Add/2

== system Model-Reglare/Model(Sis_in_bucla_deschisa)/Randament  ==
  q : Inport
  "um " : Inport  Port=2
  Gain : Gain  Gain=keta
  Product : Product
  "eta " : Outport  VectorParamsAs1DForOutWhenUnconnected=off
  wires:
  Gain/1 -> Product/2
  q/1 -> Product/1
  "um "/1 -> Gain/1
  Product/1 -> "eta "/1

== system Model-Reglare/Model(Sis_in_bucla_deschisa)/Rezervor  ==
  "qi " : Inport
  Fcn : Fcn  Expr=sqrt(u)*9
  Gain : Gain  Gain=1/332.5
  Integrator : Integrator
  Sum : Sum  Inputs=|+-
  h : Outport  VectorParamsAs1DForOutWhenUnconnected=off
  wires:
  "qi "/1 -> Sum/1
  Sum/1 -> Gain/1
  Gain/1 -> Integrator/1
  Integrator/1 -> Fcn/1, h/1
  Fcn/1 -> Sum/2

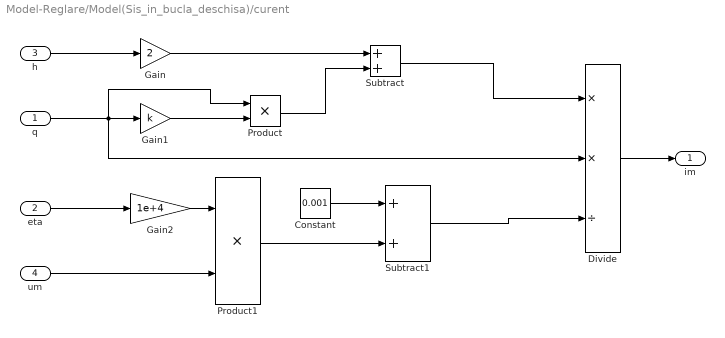
== system Model-Reglare/Model(Sis_in_bucla_deschisa)/curent  ==
  q : Inport
  eta : Inport  Port=2
  "h " : Inport  Port=3
  um : Inport  Port=4
  Constant : Constant  Value=0.001
  Divide : Product  Inputs=**/
  Gain : Gain  Gain=2
  Gain1 : Gain  Gain=k
  Gain2 : Gain  Gain=1e+4
  Product : Product
  Product1 : Product
  Subtract : Sum
  Subtract1 : Sum
  "im " : Outport  VectorParamsAs1DForOutWhenUnconnected=off
  wires:
  Constant/1 -> Subtract1/1
  Product1/1 -> Subtract1/2
  um/1 -> Product1/2
  Divide/1 -> "im "/1
  Gain2/1 -> Product1/1
  Subtract/1 -> Divide/1
  Gain1/1 -> Product/2
  eta/1 -> Gain2/1
  Product/1 -> Subtract/2
  q/1 -> Divide/2, Product/1, Gain1/1
  Subtract1/1 -> Divide/3
  Gain/1 -> Subtract/1
  "h "/1 -> Gain/1

== system Model-Reglare/Model(Sis_in_bucla_deschisa)/pompa  ==
  kn : Inport
  "h " : Inport  Port=2
  Gain : Gain  Gain=k11
  Gain1 : Gain  Gain=k2
  Gain2 : Gain  Gain=k12
  Gain3 : Gain  Gain=1/k13
  Product : Product
  Sqrt : Sqrt  SaturateOnIntegerOverflow=on
  Subtract : Sum  Inputs=+-
  Subtract1 : Sum
  "q " : Outport  VectorParamsAs1DForOutWhenUnconnected=off
  wires:
  Gain1/1 -> Subtract1/1
  Product/1 -> Gain/1
  Gain/1 -> Subtract/1
  Sqrt/1 -> Subtract1/2
  Subtract/1 -> Sqrt/1
  Gain3/1 -> "q "/1
  Gain2/1 -> Subtract/2
  Subtract1/1 -> Gain3/1
  kn/1 -> Gain1/1, Product/1, Product/2
  "h "/1 -> Gain2/1

== system Model-Reglare/PI_feed-forward/Model(Sis_in_bucla_deschisa) ==
  "ua " : Inport
  "Amplificator " : Subsystem
  "Filtru " : Subsystem
  Motor : Subsystem
  "Randament " : Subsystem
  "Rezervor " : Subsystem
  Scope : Scope
  Scope1 : Scope
  "curent " : Subsystem
  "pompa " : Subsystem
  "h " : Outport  VectorParamsAs1DForOutWhenUnconnected=off
  "Perturbatie " : Outport  Port=2  VectorParamsAs1DForOutWhenUnconnected=off
  wires:
  "ua "/1 -> "Amplificator "/1("ua ")
  "Rezervor "/1(h1) -> Scope/1, "curent "/3("h "), "pompa "/2("h "), "h "/1
  "Randament "/1("eta ") -> "curent "/2(eta)
  "pompa "/1("q ") -> "Filtru "/1("qi ")
  "Filtru "/1(q_f) -> "Rezervor "/1(q1), Scope1/1, "Randament "/1(q), "curent "/1(q)
  "Amplificator "/1("um ") -> Motor/1("um "), "Randament "/2("um "), "curent "/4(um)
  Motor/1(kn) -> "pompa "/1(kn)
  "curent "/1("im ") -> Motor/2("im ")
  "Rezervor "/2(Perturbatie1) -> "Perturbatie "/1

== system Model-Reglare/PI_perturbatie_iesire/Model_Modificat  ==
  "ua " : Inport
  "Amplificator " : Subsystem
  "Filtru " : Subsystem
  Motor : Subsystem
  "Randament " : Subsystem
  "Rezervor " : Subsystem
  Scope : Scope
  Scope1 : Scope
  "curent " : Subsystem
  "pompa " : Subsystem
  "h " : Outport  VectorParamsAs1DForOutWhenUnconnected=off
  wires:
  "ua "/1 -> "Amplificator "/1("ua ")
  "Rezervor "/1(h1) -> Scope/1, "curent "/3("h "), "pompa "/2("h "), "h "/1
  "Randament "/1("eta ") -> "curent "/2(eta)
  "pompa "/1("q ") -> "Filtru "/1("qi ")
  "Filtru "/1(q_f) -> "Rezervor "/1(q1), Scope1/1, "Randament "/1(q), "curent "/1(q)
  "Amplificator "/1("um ") -> Motor/1("um "), "Randament "/2("um "), "curent "/4(um)
  Motor/1(kn) -> "pompa "/1(kn)
  "curent "/1("im ") -> Motor/2("im ")

== system Model-Reglare/PI_perturbatie_intrare/Model_cu_perturbatie  ==
  "ua " : Inport
  "Amplificator " : Subsystem
  "Filtru " : Subsystem
  Motor : Subsystem
  "Pompa_cu_perturbatie " : Subsystem
  "Randament " : Subsystem
  "Rezervor " : Subsystem
  Scope : Scope
  Scope1 : Scope
  Step : Step  Time=250  After=0.04  SampleTime=0
  "curent " : Subsystem
  "h " : Outport  VectorParamsAs1DForOutWhenUnconnected=off
  wires:
  "ua "/1 -> "Amplificator "/1("ua ")
  "Rezervor "/1(h) -> Scope/1, "Pompa_cu_perturbatie "/2(h1), "curent "/3("h "), "h "/1
  "Randament "/1("eta ") -> "curent "/2(eta)
  "Pompa_cu_perturbatie "/1(q1) -> "Filtru "/1("qi ")
  "Filtru "/1(q_f) -> Scope1/1, "Rezervor "/1(qi), "Randament "/1(q), "curent "/1(q)
  "Amplificator "/1("um ") -> Motor/1("um "), "Randament "/2("um "), "curent "/4(um)
  Motor/1(kn) -> "Pompa_cu_perturbatie "/1(kn1)
  "curent "/1("im ") -> Motor/2("im ")
  Step/1 -> "Pompa_cu_perturbatie "/3(perturbatie k)

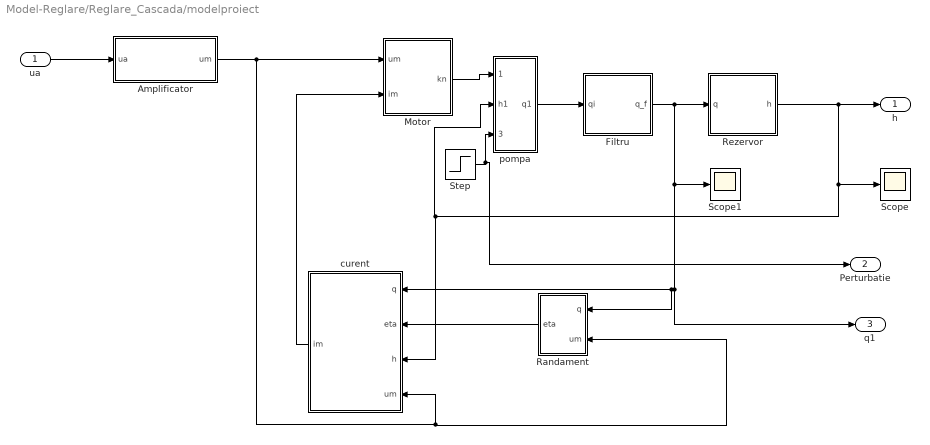
== system Model-Reglare/Reglare_Cascada/modelproiect  ==
  "ua " : Inport
  "Amplificator " : Subsystem
  "Filtru " : Subsystem
  Motor : Subsystem
  "Randament " : Subsystem
  "Rezervor " : Subsystem
  Scope : Scope
  Scope1 : Scope
  Step : Step  Time=300  After=-0.035  SampleTime=0
  "curent " : Subsystem
  "pompa " : Subsystem
  "h " : Outport  VectorParamsAs1DForOutWhenUnconnected=off
  Perturbatie : Outport  Port=2  VectorParamsAs1DForOutWhenUnconnected=off
  q1 : Outport  Port=3  VectorParamsAs1DForOutWhenUnconnected=off
  wires:
  "Amplificator "/1("um ") -> Motor/1("um "), "Randament "/2("um "), "curent "/4(um)
  "curent "/1("im ") -> Motor/2("im ")
  Step/1 -> Perturbatie/1, "pompa "/3(perturbatie k)
  "Rezervor "/1(h) -> Scope/1, "pompa "/2(h1), "curent "/3("h "), "h "/1
  "pompa "/1(q1) -> "Filtru "/1("qi ")
  "Randament "/1("eta ") -> "curent "/2(eta)
  Motor/1(kn) -> "pompa "/1(kn1)
  "Filtru "/1(q_f) -> "Rezervor "/1(q), Scope1/1, q1/1, "Randament "/1(q), "curent "/1(q)
  "ua "/1 -> "Amplificator "/1("ua ")

== system Model-Reglare/Cascada_FeedForward/modelproiect 1/Amplificator  ==
  "ua " : Inport
  Constant : Constant  Value=8.1
  Gain : Gain  Gain=2.2
  Gain1 : Gain  Gain=2.2
  Gain2 : Gain  Gain=5
  Saturation : Saturate  UpperLimit=22  LowerLimit=0
  Sum : Sum  Inputs=|+-
  Sum1 : Sum  Inputs=|++
  Switch : Switch  Criteria=u2 > Threshold  Threshold=8.1
  "um " : Outport  VectorParamsAs1DForOutWhenUnconnected=off
  wires:
  Saturation/1 -> "um "/1
  Switch/1 -> Saturation/1
  Constant/1 -> Sum/2
  Sum/1 -> Gain2/1
  Sum1/1 -> Switch/1
  Gain1/1 -> Sum1/1
  Gain/1 -> Switch/3
  "ua "/1 -> Switch/2, Gain/1, Sum/1, Gain1/1
  Gain2/1 -> Sum1/2

== system Model-Reglare/Cascada_FeedForward/modelproiect 1/Filtru  ==
  "qi " : Inport
  Integrator : Integrator  InitialCondition=29.2
  Sum : Sum  Inputs=|+-
  q_f : Outport  VectorParamsAs1DForOutWhenUnconnected=off
  wires:
  "qi "/1 -> Sum/1
  Sum/1 -> Integrator/1
  Integrator/1 -> Sum/2, q_f/1

== system Model-Reglare/Cascada_FeedForward/modelproiect 1/Motor ==
  "um " : Inport
  "im " : Inport  Port=2
  Add : Sum  Inputs=+-
  Rm : Gain  Gain=3
  kn : Outport  VectorParamsAs1DForOutWhenUnconnected=off
  wires:
  "um "/1 -> Add/1
  "im "/1 -> Rm/1
  Add/1 -> kn/1
  Rm/1 -> Add/2

== system Model-Reglare/Cascada_FeedForward/modelproiect 1/Randament  ==
  q : Inport
  "um " : Inport  Port=2
  Gain : Gain  Gain=keta
  Product : Product
  "eta " : Outport  VectorParamsAs1DForOutWhenUnconnected=off
  wires:
  Gain/1 -> Product/2
  q/1 -> Product/1
  "um "/1 -> Gain/1
  Product/1 -> "eta "/1

== system Model-Reglare/Cascada_FeedForward/modelproiect 1/Rezervor 1 ==
  q1 : Inport
  Add1 : Sum
  C1 : Constant  Value=9
  Gain1 : Gain  Gain=1/332.5
  Integrator1 : Integrator  InitialCondition=10.5
  Product3 : Product
  Product4 : Product
  Scope1 : Scope
  Sqrt2 : Sqrt  IntermediateResultsDataTypeStr=double  SaturateOnIntegerOverflow=on
  Step1 : Step  Time=500  After=2  SampleTime=0
  Sum1 : Sum  Inputs=|+-
  h1 : Outport  VectorParamsAs1DForOutWhenUnconnected=off
  Perturbatie1 : Outport  Port=2  VectorParamsAs1DForOutWhenUnconnected=off
  wires:
  Sqrt2/1 -> Product3/1, Product4/1
  Product3/1 -> Scope1/1, Sum1/2
  Step1/1 -> Product4/2, Add1/1
  Product4/1 -> Perturbatie1/1
  Integrator1/1 -> Sqrt2/1, h1/1
  C1/1 -> Add1/2
  Gain1/1 -> Integrator1/1
  Sum1/1 -> Gain1/1
  q1/1 -> Sum1/1
  Add1/1 -> Product3/2

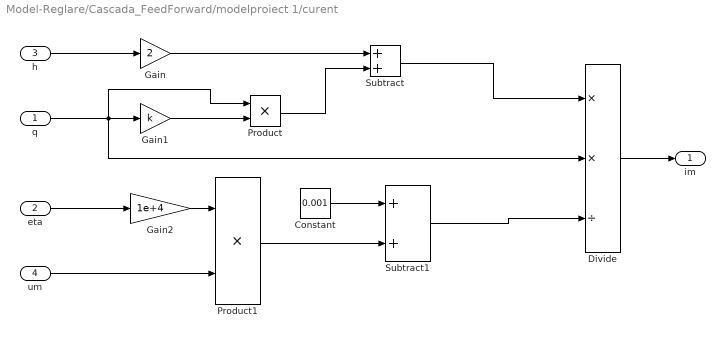
== system Model-Reglare/Cascada_FeedForward/modelproiect 1/curent  ==
  q : Inport
  eta : Inport  Port=2
  "h " : Inport  Port=3
  um : Inport  Port=4
  Constant : Constant  Value=0.001
  Divide : Product  Inputs=**/
  Gain : Gain  Gain=2
  Gain1 : Gain  Gain=k
  Gain2 : Gain  Gain=1e+4
  Product : Product
  Product1 : Product
  Subtract : Sum
  Subtract1 : Sum
  "im " : Outport  VectorParamsAs1DForOutWhenUnconnected=off
  wires:
  Constant/1 -> Subtract1/1
  Product1/1 -> Subtract1/2
  um/1 -> Product1/2
  Divide/1 -> "im "/1
  Gain2/1 -> Product1/1
  Subtract/1 -> Divide/1
  Gain1/1 -> Product/2
  eta/1 -> Gain2/1
  Product/1 -> Subtract/2
  q/1 -> Divide/2, Product/1, Gain1/1
  Subtract1/1 -> Divide/3
  Gain/1 -> Subtract/1
  "h "/1 -> Gain/1

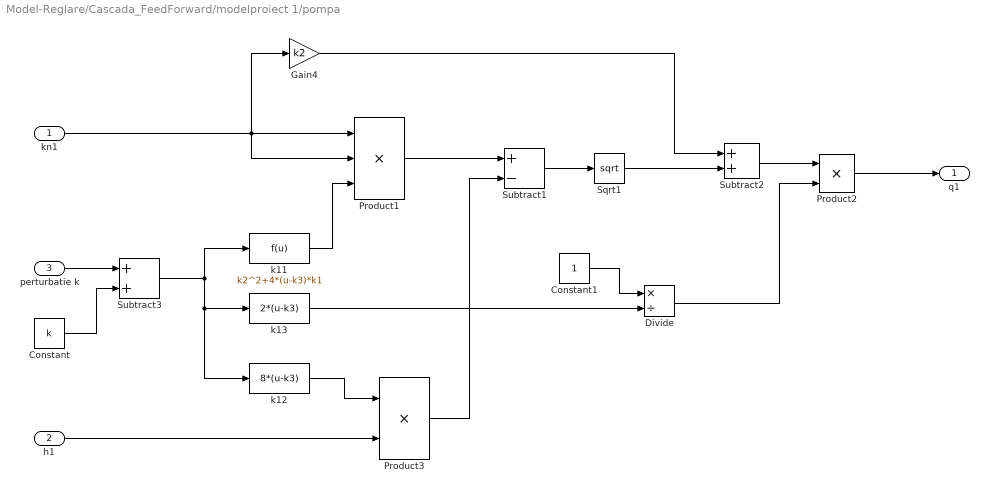
== system Model-Reglare/Cascada_FeedForward/modelproiect 1/pompa  ==
  kn1 : Inport
  h1 : Inport  Port=2
  perturbatie k : Inport  Port=3
  Constant : Constant  Value=k
  Constant1 : Constant
  Divide : Product  Inputs=*/
  Gain4 : Gain  Gain=k2
  Product1 : Product  Inputs=3
  Product2 : Product
  Product3 : Product
  Sqrt1 : Sqrt  SaturateOnIntegerOverflow=on
  Subtract1 : Sum  Inputs=+-
  Subtract2 : Sum
  Subtract3 : Sum
  k11 : Fcn  Expr=k2^2+4*(u-k3)*k1
  k12 : Fcn  Expr=8*(u-k3)
  k13 : Fcn  Expr=2*(u-k3)
  q1 : Outport  VectorParamsAs1DForOutWhenUnconnected=off
  wires:
  Constant1/1 -> Divide/1
  Subtract2/1 -> Product2/1
  Product2/1 -> q1/1
  Subtract1/1 -> Sqrt1/1
  perturbatie k/1 -> Subtract3/1
  Divide/1 -> Product2/2
  Gain4/1 -> Subtract2/1
  Product1/1 -> Subtract1/1
  k11/1 -> Product1/3
  k13/1 -> Divide/2
  Sqrt1/1 -> Subtract2/2
  Constant/1 -> Subtract3/2
  k12/1 -> Product3/1
  Product3/1 -> Subtract1/2
  Subtract3/1 -> k12/1, k13/1, k11/1
  h1/1 -> Product3/2
  kn1/1 -> Gain4/1, Product1/1, Product1/2

== system Model-Reglare/Fara_Perturbatie/Sistem in bucla deschisa 1/Amplificator  ==
  "ua " : Inport
  Constant : Constant  Value=8.1
  Gain : Gain  Gain=2.2
  Gain1 : Gain  Gain=2.2
  Gain2 : Gain  Gain=5
  Saturation : Saturate  UpperLimit=22  LowerLimit=0
  Sum : Sum  Inputs=|+-
  Sum1 : Sum  Inputs=|++
  Switch : Switch  Criteria=u2 > Threshold  Threshold=8.1
  "um " : Outport  VectorParamsAs1DForOutWhenUnconnected=off
  wires:
  Saturation/1 -> "um "/1
  Switch/1 -> Saturation/1
  Constant/1 -> Sum/2
  Sum/1 -> Gain2/1
  Sum1/1 -> Switch/1
  Gain1/1 -> Sum1/1
  Gain/1 -> Switch/3
  "ua "/1 -> Switch/2, Gain/1, Sum/1, Gain1/1
  Gain2/1 -> Sum1/2

== system Model-Reglare/Fara_Perturbatie/Sistem in bucla deschisa 1/Filtru  ==
  "qi " : Inport
  Integrator : Integrator  InitialCondition=29.2
  Sum : Sum  Inputs=|+-
  q_f : Outport  VectorParamsAs1DForOutWhenUnconnected=off
  wires:
  "qi "/1 -> Sum/1
  Sum/1 -> Integrator/1
  Integrator/1 -> Sum/2, q_f/1

== system Model-Reglare/Fara_Perturbatie/Sistem in bucla deschisa 1/Motor ==
  "um " : Inport
  "im " : Inport  Port=2
  Add : Sum  Inputs=+-
  Rm : Gain  Gain=3
  kn : Outport  VectorParamsAs1DForOutWhenUnconnected=off
  wires:
  "um "/1 -> Add/1
  "im "/1 -> Rm/1
  Add/1 -> kn/1
  Rm/1 -> Add/2

== system Model-Reglare/Fara_Perturbatie/Sistem in bucla deschisa 1/Randament  ==
  q : Inport
  "um " : Inport  Port=2
  Gain : Gain  Gain=keta
  Product : Product
  "eta " : Outport  VectorParamsAs1DForOutWhenUnconnected=off
  wires:
  Gain/1 -> Product/2
  q/1 -> Product/1
  "um "/1 -> Gain/1
  Product/1 -> "eta "/1

== system Model-Reglare/Fara_Perturbatie/Sistem in bucla deschisa 1/Rezervor  ==
  "qi " : Inport
  Fcn : Fcn  Expr=sqrt(u)*9
  Gain : Gain  Gain=1/332.5
  Integrator : Integrator  InitialCondition=10.5
  Sum : Sum  Inputs=|+-
  h : Outport  VectorParamsAs1DForOutWhenUnconnected=off
  wires:
  "qi "/1 -> Sum/1
  Sum/1 -> Gain/1
  Gain/1 -> Integrator/1
  Integrator/1 -> Fcn/1, h/1
  Fcn/1 -> Sum/2

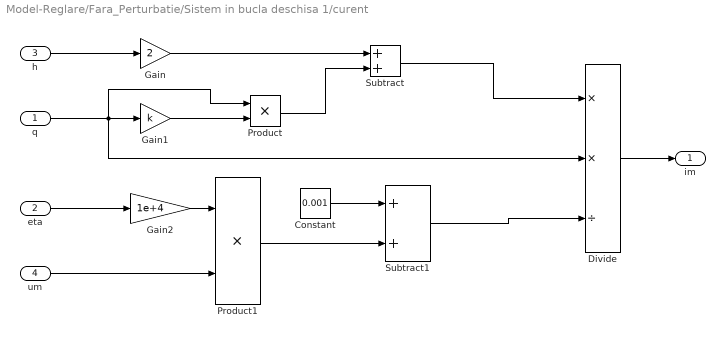
== system Model-Reglare/Fara_Perturbatie/Sistem in bucla deschisa 1/curent  ==
  q : Inport
  eta : Inport  Port=2
  "h " : Inport  Port=3
  um : Inport  Port=4
  Constant : Constant  Value=0.001
  Divide : Product  Inputs=**/
  Gain : Gain  Gain=2
  Gain1 : Gain  Gain=k
  Gain2 : Gain  Gain=1e+4
  Product : Product
  Product1 : Product
  Subtract : Sum
  Subtract1 : Sum
  "im " : Outport  VectorParamsAs1DForOutWhenUnconnected=off
  wires:
  Constant/1 -> Subtract1/1
  Product1/1 -> Subtract1/2
  um/1 -> Product1/2
  Divide/1 -> "im "/1
  Gain2/1 -> Product1/1
  Subtract/1 -> Divide/1
  Gain1/1 -> Product/2
  eta/1 -> Gain2/1
  Product/1 -> Subtract/2
  q/1 -> Divide/2, Product/1, Gain1/1
  Subtract1/1 -> Divide/3
  Gain/1 -> Subtract/1
  "h "/1 -> Gain/1

== system Model-Reglare/Fara_Perturbatie/Sistem in bucla deschisa 1/pompa  ==
  kn : Inport
  "h " : Inport  Port=2
  Gain : Gain  Gain=k11
  Gain1 : Gain  Gain=k2
  Gain2 : Gain  Gain=k12
  Gain3 : Gain  Gain=1/k13
  Product : Product
  Sqrt : Sqrt  SaturateOnIntegerOverflow=on
  Subtract : Sum  Inputs=+-
  Subtract1 : Sum
  "q " : Outport  VectorParamsAs1DForOutWhenUnconnected=off
  wires:
  Gain1/1 -> Subtract1/1
  Product/1 -> Gain/1
  Gain/1 -> Subtract/1
  Sqrt/1 -> Subtract1/2
  Subtract/1 -> Sqrt/1
  Gain3/1 -> "q "/1
  Gain2/1 -> Subtract/2
  Subtract1/1 -> Gain3/1
  kn/1 -> Gain1/1, Product/1, Product/2
  "h "/1 -> Gain2/1

== system Model-Reglare/PI_feed-forward/Model(Sis_in_bucla_deschisa)/Amplificator  ==
  "ua " : Inport
  Constant : Constant  Value=8.1
  Gain : Gain  Gain=2.2
  Gain1 : Gain  Gain=2.2
  Gain2 : Gain  Gain=5
  Saturation : Saturate  UpperLimit=22  LowerLimit=0
  Sum : Sum  Inputs=|+-
  Sum1 : Sum  Inputs=|++
  Switch : Switch  Criteria=u2 > Threshold  Threshold=8.1
  "um " : Outport  VectorParamsAs1DForOutWhenUnconnected=off
  wires:
  Saturation/1 -> "um "/1
  Switch/1 -> Saturation/1
  Constant/1 -> Sum/2
  Sum/1 -> Gain2/1
  Sum1/1 -> Switch/1
  Gain1/1 -> Sum1/1
  Gain/1 -> Switch/3
  "ua "/1 -> Switch/2, Gain/1, Sum/1, Gain1/1
  Gain2/1 -> Sum1/2

== system Model-Reglare/PI_feed-forward/Model(Sis_in_bucla_deschisa)/Filtru  ==
  "qi " : Inport
  Integrator : Integrator  InitialCondition=29.2
  Sum : Sum  Inputs=|+-
  q_f : Outport  VectorParamsAs1DForOutWhenUnconnected=off
  wires:
  "qi "/1 -> Sum/1
  Sum/1 -> Integrator/1
  Integrator/1 -> Sum/2, q_f/1

== system Model-Reglare/PI_feed-forward/Model(Sis_in_bucla_deschisa)/Motor ==
  "um " : Inport
  "im " : Inport  Port=2
  Add : Sum  Inputs=+-
  Rm : Gain  Gain=3
  kn : Outport  VectorParamsAs1DForOutWhenUnconnected=off
  wires:
  "um "/1 -> Add/1
  "im "/1 -> Rm/1
  Add/1 -> kn/1
  Rm/1 -> Add/2

== system Model-Reglare/PI_feed-forward/Model(Sis_in_bucla_deschisa)/Randament  ==
  q : Inport
  "um " : Inport  Port=2
  Gain : Gain  Gain=keta
  Product : Product
  "eta " : Outport  VectorParamsAs1DForOutWhenUnconnected=off
  wires:
  Gain/1 -> Product/2
  q/1 -> Product/1
  "um "/1 -> Gain/1
  Product/1 -> "eta "/1

== system Model-Reglare/PI_feed-forward/Model(Sis_in_bucla_deschisa)/Rezervor  ==
  q1 : Inport
  Add1 : Sum
  C1 : Constant  Value=9
  Gain1 : Gain  Gain=1/332.5
  Integrator1 : Integrator  InitialCondition=10.5
  Product3 : Product
  Product4 : Product
  Scope1 : Scope
  Sqrt2 : Sqrt  IntermediateResultsDataTypeStr=double  SaturateOnIntegerOverflow=on
  Step1 : Step  Time=500  After=2  SampleTime=0
  Sum1 : Sum  Inputs=|+-
  h1 : Outport  VectorParamsAs1DForOutWhenUnconnected=off
  Perturbatie1 : Outport  Port=2  VectorParamsAs1DForOutWhenUnconnected=off
  wires:
  Sqrt2/1 -> Product3/1, Product4/1
  Product3/1 -> Scope1/1, Sum1/2
  Step1/1 -> Product4/2, Add1/1
  Product4/1 -> Perturbatie1/1
  Integrator1/1 -> Sqrt2/1, h1/1
  C1/1 -> Add1/2
  Gain1/1 -> Integrator1/1
  Sum1/1 -> Gain1/1
  q1/1 -> Sum1/1
  Add1/1 -> Product3/2

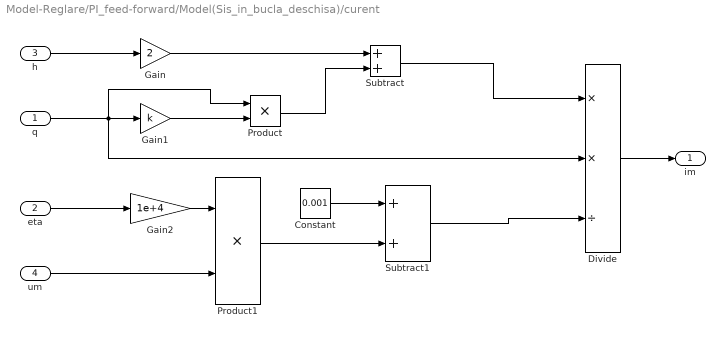
== system Model-Reglare/PI_feed-forward/Model(Sis_in_bucla_deschisa)/curent  ==
  q : Inport
  eta : Inport  Port=2
  "h " : Inport  Port=3
  um : Inport  Port=4
  Constant : Constant  Value=0.001
  Divide : Product  Inputs=**/
  Gain : Gain  Gain=2
  Gain1 : Gain  Gain=k
  Gain2 : Gain  Gain=1e+4
  Product : Product
  Product1 : Product
  Subtract : Sum
  Subtract1 : Sum
  "im " : Outport  VectorParamsAs1DForOutWhenUnconnected=off
  wires:
  Constant/1 -> Subtract1/1
  Product1/1 -> Subtract1/2
  um/1 -> Product1/2
  Divide/1 -> "im "/1
  Gain2/1 -> Product1/1
  Subtract/1 -> Divide/1
  Gain1/1 -> Product/2
  eta/1 -> Gain2/1
  Product/1 -> Subtract/2
  q/1 -> Divide/2, Product/1, Gain1/1
  Subtract1/1 -> Divide/3
  Gain/1 -> Subtract/1
  "h "/1 -> Gain/1

== system Model-Reglare/PI_feed-forward/Model(Sis_in_bucla_deschisa)/pompa  ==
  kn : Inport
  "h " : Inport  Port=2
  Gain : Gain  Gain=k11
  Gain1 : Gain  Gain=k2
  Gain2 : Gain  Gain=k12
  Gain3 : Gain  Gain=1/k13
  Product : Product
  Sqrt : Sqrt  SaturateOnIntegerOverflow=on
  Subtract : Sum  Inputs=+-
  Subtract1 : Sum
  "q " : Outport  VectorParamsAs1DForOutWhenUnconnected=off
  wires:
  Gain1/1 -> Subtract1/1
  Product/1 -> Gain/1
  Gain/1 -> Subtract/1
  Sqrt/1 -> Subtract1/2
  Subtract/1 -> Sqrt/1
  Gain3/1 -> "q "/1
  Gain2/1 -> Subtract/2
  Subtract1/1 -> Gain3/1
  kn/1 -> Gain1/1, Product/1, Product/2
  "h "/1 -> Gain2/1
